simulink model "FAULTMODEL"  (R2024a)
settings: Solver=VariableStepAuto  StartTime=0.0  StopTime=0.08  RelTol=1e-3
libraries: spsThreePhaseVIMeasurementLib x4, spsThreePhaseSourceLib x2, spsThreePhasePISectionLineLib x2, spsThreePhaseParallelRLCLoadLib x1, spsThreePhaseFaultLib x1, sps_lib x1
settings Model: Creator=hp  LastModifiedBy=plali
settings RTWCC: GPUComputeCapability=3.5

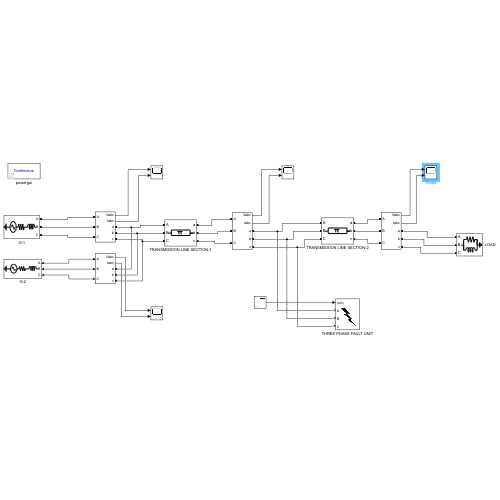
[thumbnail: Simulink's stored preview of the top-level diagram]
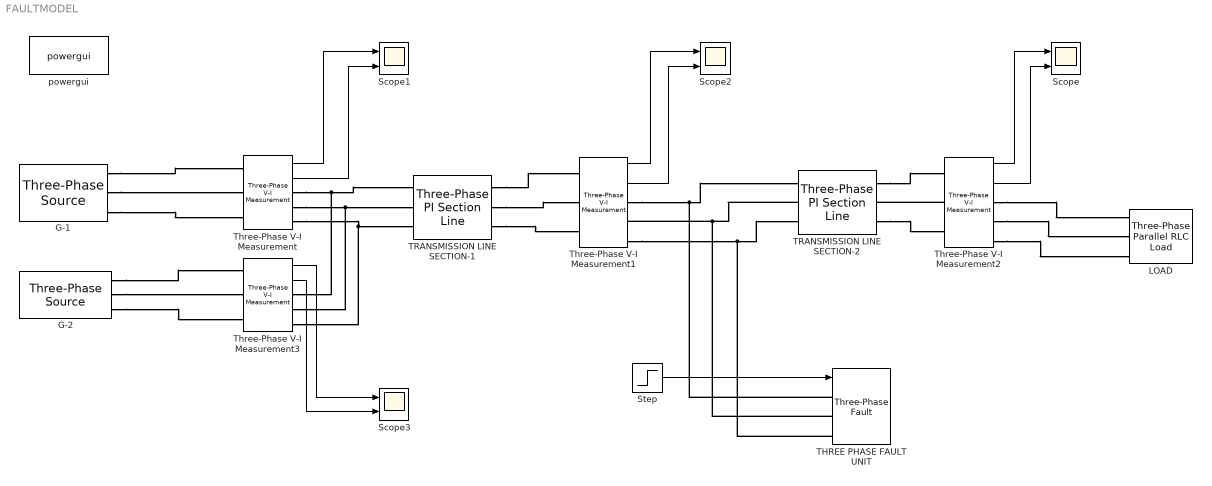
== system FAULTMODEL ==
  G-1 : spsThreePhaseSourceLib/Three-Phase Source  InternalConnection=Yg  VoltagePhases=off  Voltage=25e3  PhaseAngle=0  Voltage_phases=[25e3 25e3 25e3]/sqrt(3)  PhaseAngles_phases=[0 -120 +120]  Frequency=50  NonIdealSource=on  SpecifyImpedance=off  Resistance=0.8929  Inductance=16.58e-3  ShortCircuitLevel=100e6  BaseVoltage=25e3  XRratio=7  BusType=swing  Pref=10e3  Qref=0  Prefabc=[10e3, 10e3, 10e3]  Qrefabc=[0, 0, 0]  Qmin=-inf  Qmax=inf
  G-2 : spsThreePhaseSourceLib/Three-Phase Source  InternalConnection=Yg  VoltagePhases=off  Voltage=25e3  PhaseAngle=0  Voltage_phases=[25e3 25e3 25e3]/sqrt(3)  PhaseAngles_phases=[0 -120 +120]  Frequency=50  NonIdealSource=on  SpecifyImpedance=off  Resistance=10  Inductance=16.58e-3  ShortCircuitLevel=100e6  BaseVoltage=25e3  XRratio=7  BusType=swing  Pref=10e3  Qref=0  Prefabc=[10e3, 10e3, 10e3]  Qrefabc=[0, 0, 0]  Qmin=-inf  Qmax=inf
  LOAD : spsThreePhaseParallelRLCLoadLib/Three-Phase Parallel RLC Load  LConnTagsString=A|B|C  Configuration=Y (grounded)  NominalVoltage=1000  Vabc=[1e3 1e3 1e3]  Vabcp=[1e3 1e3 1e3]  NominalFrequency=50  UnbalancedPower=off  ActivePower=10e3  InductivePower=100  CapacitivePower=0  Pabc=[10e3 9e3 11e3]  QLabc=[100 90 110]  QCabc=[100 90 110]  Pabcp=[10e3 9e3 11e3]  QLabcp=[100 90 110]  QCabcp=[100 90 110]  Measurements=None  LoadType=constant Z
  Scope{,1..3} (4 alike) : Scope  NumInputPorts=2
  Step : Step  Time=0.04  SampleTime=0
  THREE PHASE FAULT UNIT : spsThreePhaseFaultLib/Three-Phase Fault  InitialStates=0  FaultA=on  FaultB=on  FaultC=on  GroundFault=off  SwitchTimes=[5.02/50]  External=on  SwitchStatus=NaN  FaultResistance=0.005  GroundResistance=0.1  SnubberResistance=1e6  SnubberCapacitance=inf  Measurements=None
  TRANSMISSION LINE SECTION-1 : spsThreePhasePISectionLineLib/Three-Phase PI Section Line  LConnTagsString=a|b|c  RConnTagsString=A|B|C  Length=10  Frequency=50  Resistances=[ 0.01273 0.3864]  Inductances="[ 0.9337e-3  4.1264e-3]"  Capacitances=[12.74e-9 7.751e-9]
  TRANSMISSION LINE SECTION-2 : spsThreePhasePISectionLineLib/Three-Phase PI Section Line  LConnTagsString=a|b|c  RConnTagsString=A|B|C  Length=70  Frequency=50  Resistances=[ 0.01273 0.3864]  Inductances="[ 0.9337e-3  4.1264e-3]"  Capacitances=[12.74e-9 7.751e-9]
  Three-Phase V-I Measurement{,1..3} (4 alike) : spsThreePhaseVIMeasurementLib/Three-Phase V-I Measurement  VoltageMeasurement=phase-to-ground  SetLabelV=off  LabelV=Vabc  Vpu=off  VpuLL=off  CurrentMeasurement=yes  SetLabelI=off  LabelI=Iabc  Ipu=off  Pbase=100e6  Vbase=500e3  OutputType=Complex  PhasorSimulation=off  PSBequivalent=0
  powergui : sps_lib/powergui  Priority=1  SimulationMode=Continuous  SampleTime=50e-6  frequency=60  Iterations=50  frequencyindice=50  Pbase=100e6  ErrMax=1e-4  UnitsV=kV  UnitsW=MW  buscounter=0  FunctionMessages=off  echomessages=off  EnableUseOfTLC=off  CurrentSourceSwitches=off  DisableSnubberDevices=off  DisableRonSwitches=off  DisableVfSwitches=off  DisplayEquations=off  AutomaticDiscreteSolvers=off  SolverType=Tustin/Backward Euler (TBE)  Interpol=off  ExternalGateDelay=off  methode=off  Ts=100  x0status=blocks  SPID=on  SwTol=0  HookPort=off  NonlinearTolerance=1e-4  nMaxIteration=100  ContinueOnMaxIteration=off  RestoreLinks=warning  ResistiveCurrentMeasurement=off  Frange=[0:2:500]  Ylog=off  Xlog=on  ShowGrid=off  save=off  variable=ZData  structure=0  ZoomFFT=off  StartTime=0.0  cycles=1  DisplayStyle=1  fundamental=60  FreqAxis=off  MaxFrequency=1000  frequencyindicesteady=1  RmsSteady=1  display=off
  wires:
  Three-Phase V-I Measurement/1 -> Scope1/1
  Three-Phase V-I Measurement/2 -> Scope1/2
  Three-Phase V-I Measurement1/1 -> Scope2/1
  Three-Phase V-I Measurement1/2 -> Scope2/2
  Three-Phase V-I Measurement2/1 -> Scope/1
  Three-Phase V-I Measurement2/2 -> Scope/2
  Three-Phase V-I Measurement3/1 -> Scope3/1
  Three-Phase V-I Measurement3/2 -> Scope3/2
  Step/1 -> THREE PHASE FAULT UNIT/1
  connections:
  G-1/RConn1 -- Three-Phase V-I Measurement/LConn1
  G-1/RConn2 -- Three-Phase V-I Measurement/LConn2
  G-1/RConn3 -- Three-Phase V-I Measurement/LConn3
  G-2/RConn2 -- Three-Phase V-I Measurement3/LConn2
  G-2/RConn1 -- Three-Phase V-I Measurement3/LConn1
  G-2/RConn3 -- Three-Phase V-I Measurement3/LConn3
  Three-Phase V-I Measurement/RConn1 -- Three-Phase V-I Measurement3/RConn1 -- TRANSMISSION LINE SECTION-1/LConn1
  Three-Phase V-I Measurement/RConn2 -- Three-Phase V-I Measurement3/RConn2 -- TRANSMISSION LINE SECTION-1/LConn2
  Three-Phase V-I Measurement/RConn3 -- Three-Phase V-I Measurement3/RConn3 -- TRANSMISSION LINE SECTION-1/LConn3
  TRANSMISSION LINE SECTION-1/RConn1 -- Three-Phase V-I Measurement1/LConn1
  TRANSMISSION LINE SECTION-1/RConn2 -- Three-Phase V-I Measurement1/LConn2
  TRANSMISSION LINE SECTION-1/RConn3 -- Three-Phase V-I Measurement1/LConn3
  TRANSMISSION LINE SECTION-2/LConn2 -- THREE PHASE FAULT UNIT/LConn2 -- Three-Phase V-I Measurement1/RConn2
  Three-Phase V-I Measurement1/RConn1 -- THREE PHASE FAULT UNIT/LConn1 -- TRANSMISSION LINE SECTION-2/LConn1
  Three-Phase V-I Measurement1/RConn3 -- THREE PHASE FAULT UNIT/LConn3 -- TRANSMISSION LINE SECTION-2/LConn3
  Three-Phase V-I Measurement2/LConn2 -- TRANSMISSION LINE SECTION-2/RConn2
  TRANSMISSION LINE SECTION-2/RConn1 -- Three-Phase V-I Measurement2/LConn1
  TRANSMISSION LINE SECTION-2/RConn3 -- Three-Phase V-I Measurement2/LConn3
  Three-Phase V-I Measurement2/RConn1 -- LOAD/LConn1
  Three-Phase V-I Measurement2/RConn2 -- LOAD/LConn2
  Three-Phase V-I Measurement2/RConn3 -- LOAD/LConn3
